simulink subsystem "EKF"  (R2022b)
settings: Solver=VariableStepAuto  StartTime=0.0  StopTime=10.0  RelTol=1e-3
model mask{motor_model=0, Q=0, R=0, Ts=-1}
  mask prompts: motor_model "System Model:"; Q "Process Noise Variance (Q):"; R "Measurement Noise Variance (R):"; Ts "Sampling Time:"
undefined symbols (not defined in the file): nl_options
libraries: sharedTrackingLibrary x1
settings Model: Creator=gotta  LastModifiedBy=gotta

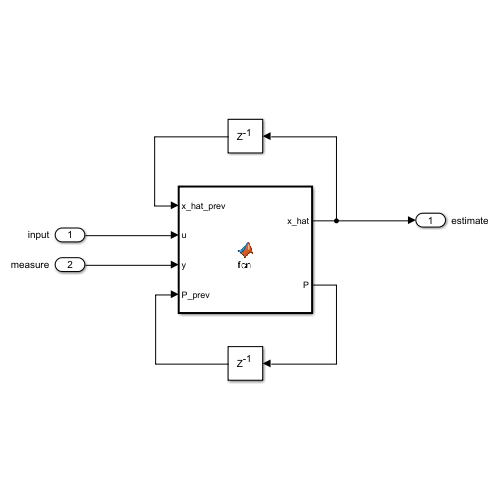
[thumbnail: Simulink's stored preview of the top-level diagram]
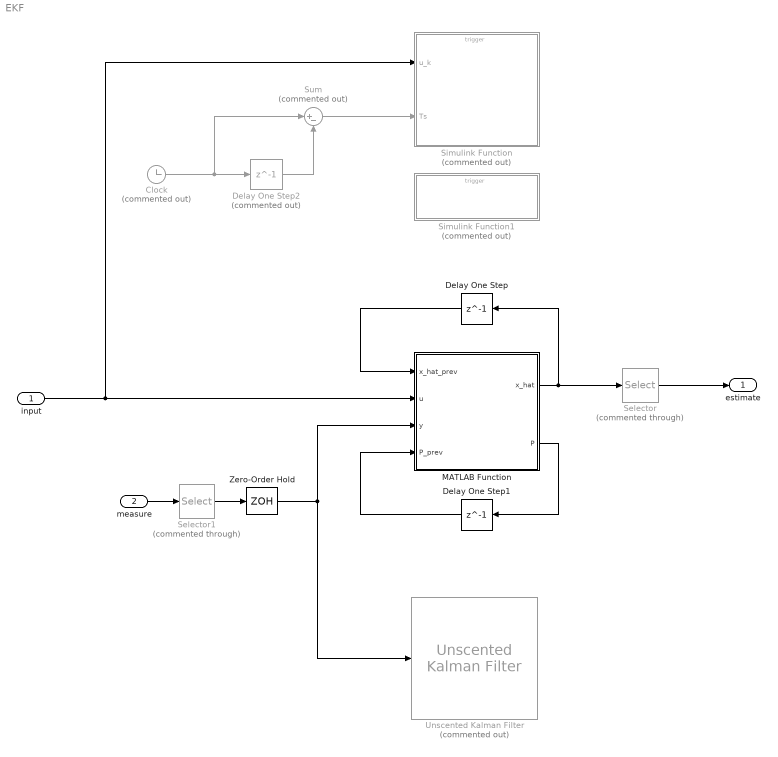
== system EKF ==
  input : Inport
  measure : Inport  Port=2
  Clock : Clock  Commented=on
  Delay One Step : Delay  DelayLength=1  InitialCondition=zeros(4,1)  SampleTime=Ts
  Delay One Step1 : Delay  DelayLength=1  InitialCondition=1e-2*eye(4)  SampleTime=Ts
  Delay One Step2 : Delay  Commented=on  DelayLength=1
  MATLAB Function : MATLAB Function  TreatAsAtomicUnit=on
  Selector : Selector  Commented=through  InputPortWidth=4  IndexOptions=Index vector (dialog)  Indices=[1:3]  OutputSizes=1
  Selector1 : Selector  Commented=through  InputPortWidth=3  IndexOptions=Index vector (dialog)  Indices=[1 3]  OutputSizes=1
  Simulink Function : Subsystem  Commented=on  TreatAsAtomicUnit=on
  Simulink Function1 : Subsystem  Commented=on  TreatAsAtomicUnit=on
  Sum : Sum  Commented=on  Inputs=|+-
  Unscented Kalman Filter : sharedTrackingLibrary/Unscented Kalman Filter  Commented=on  StateTransitionFcn=model_dynamics  HasAdditiveProcessNoise=Additive  ProcessNoise=Q  HasTimeVaryingProcessNoise=off  HasStateTransitionFcnExtraArgument=0  InitialState=zeros(4,1)  InitialStateCovariance=1e-6*eye(4)  Alpha=1e-3  Beta=2  Kappa=0  MeasurementFcn1=state_measurement  HasMeasurementEnablePort1=off  HasAdditiveMeasurementNoise1=Additive  MeasurementNoise1=R  HasTimeVaryingMeasurementNoise1=off  HasMeasurementFcnExtraArgument1=0  HasMeasurementWrapping1=off  MeasurementFcn2=1  HasMeasurementEnablePort2=off  HasAdditiveMeasurementNoise2=Additive  MeasurementNoise2=1  HasTimeVaryingMeasurementNoise2=off  HasMeasurementFcnExtraArgument2=0  HasMeasurementWrapping2=off  MeasurementFcn3=myMeasurementFcn  HasMeasurementEnablePort3=off  HasAdditiveMeasurementNoise3=Additive  MeasurementNoise3=1  HasTimeVaryingMeasurementNoise3=off  HasMeasurementFcnExtraArgument3=0  HasMeasurementWrapping3=off  MeasurementFcn4=myMeasurementFcn  HasMeasurementEnablePort4=off  HasAdditiveMeasurementNoise4=Additive  MeasurementNoise4=1  HasTimeVaryingMeasurementNoise4=off  HasMeasurementFcnExtraArgument4=0  HasMeasurementWrapping4=off  MeasurementFcn5=myMeasurementFcn  HasMeasurementEnablePort5=off  HasAdditiveMeasurementNoise5=Additive  MeasurementNoise5=1  HasTimeVaryingMeasurementNoise5=off  HasMeasurementFcnExtraArgument5=0  HasMeasurementWrapping5=off  EnableMultirate=off  StateTransitionFcnSampleTime=1  MeasurementFcn1SampleTime=1  MeasurementFcn2SampleTime=1  MeasurementFcn3SampleTime=1  MeasurementFcn4SampleTime=1  MeasurementFcn5SampleTime=1  UseCurrentEstimator=on  OutputStateCovariance=off  DataType=double  SampleTime=Ts  NumberOfMeasurements=1
      settings: LibrarySourceBlock=cstblocks/State Estimation/Unscented Kalman Filter
  Zero-Order Hold : ZeroOrderHold  SampleTime=Ts
  estimate : Outport
  wires:
  measure/1 -> Selector1/1
  Delay One Step/1 -> MATLAB Function/1(x_hat_prev)
  MATLAB Function/2(P) -> Delay One Step1/1
  Delay One Step1/1 -> MATLAB Function/4(P_prev)
  Selector/1 -> estimate/1
  MATLAB Function/1(x_hat) -> Delay One Step/1, Selector/1
  Selector1/1 -> Zero-Order Hold/1
  Zero-Order Hold/1 -> Unscented Kalman Filter/1, MATLAB Function/3(y)
  input/1 -> MATLAB Function/2(u), Simulink Function/1(u_k)
  Clock/1 -> Delay One Step2/1, Sum/1
  Delay One Step2/1 -> Sum/2
  Sum/1 -> Simulink Function/2(Ts)

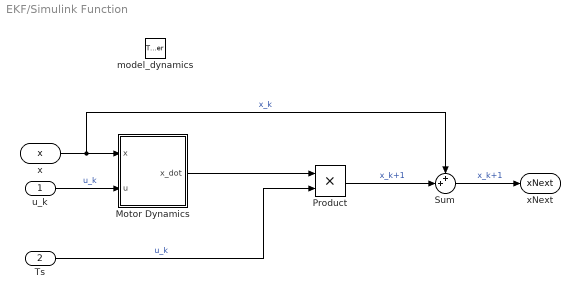
== system EKF/Simulink Function ==
  u_k : Inport
  Ts : Inport  Port=2
  model_dynamics : TriggerPort  TriggerType=function-call  IsSimulinkFunction=on  FunctionName=model_dynamics  FunctionVisibility=scoped  VariantControl=(inherit)
  Motor Dynamics : MATLAB Function  TreatAsAtomicUnit=on
  Product : Product
  Sum : Sum  Inputs=++|
  x : ArgIn  DisableCoverage=on  PortDimensions=4  ArgumentName=x
  xNext : ArgOut  DisableCoverage=on  PortDimensions=4  ArgumentName=xNext
  wires:
  Ts/1 -> Product/2  "u_k"
  Sum/1 -> xNext/1  "x_k+1"
  Motor Dynamics/1(x_dot) -> Product/1
  Product/1 -> Sum/2  "x_k+1"
  u_k/1 -> Motor Dynamics/2(u)  "u_k"
  x/1 -> Motor Dynamics/1(x), Sum/1  "x_k"

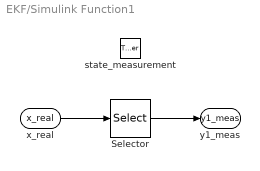
== system EKF/Simulink Function1 ==
  state_measurement : TriggerPort  TriggerType=function-call  IsSimulinkFunction=on  FunctionName=state_measurement  FunctionVisibility=scoped  VariantControl=(inherit)
  Selector : Selector  InputPortWidth=4  IndexOptions=Index vector (dialog)  Indices=[1:3]  OutputSizes=1
  x_real : ArgIn  DisableCoverage=on  PortDimensions=4  ArgumentName=x_real
  y1_meas : ArgOut  DisableCoverage=on  PortDimensions=3  ArgumentName=y1_meas
  wires:
  Selector/1 -> y1_meas/1
  x_real/1 -> Selector/1

== matlab function EKF/MATLAB Function ==
  data: x_hat_prev input; u input; x_hat output; y input; P_prev input; P output; Q parameter; R parameter; Ts parameter; motor_model parameter; nl_options parameter
function [x_hat, P] = fcn(x_hat_prev, u, y, P_prev, Q, R, Ts, motor_model, nl_options)

% Discrete step advance
x_dot = motor_dynamics(x_hat_prev, u, motor_model, nl_options);
F = motor_jacobian(x_hat_prev, motor_model, nl_options);

x_hat_pred = x_hat_prev + Ts * x_dot;


% Covariance
P_pred = F  * P_prev * transpose(F) + Q;


% Measure model
H = [1,0,0,0; 0,1,0,0; 0,0,1,0];
y_pred = H * x_hat_pred;


% Update
y_tilda = y - y_pred;
S = H * P_pred * transpose(H) + R;
K = P_pred * transpose(H) * pinv(S);
x_upd = x_hat_pred + K * y_tilda;
P_upd = (eye(4) - K * H) * P_pred;


% Output
x_hat = x_upd;
P = P_upd;

== matlab function EKF/Simulink Function/Motor Dynamics ==
  data: x input; u input; x_dot output; motor_model parameter
function x_dot = fcn(x, u, motor_model)

% Motor Dynamics

nl_options.flux = 0;
nl_options.coulomb = 0;
nl_options.stribeck = 0;

x_dot = motor_dynamics(x, u, motor_model, nl_options);
